simulink model "SESS_PassiveModel"  (R2018b)
settings: Solver=VariableStepAuto  StartTime=0.0  StopTime=1400  MaxStep=0.01  MinStep=0.00005  RelTol=1e-3
libraries: powerlib x4, electricdrivelib x1
settings Model: Creator=ttran  LastModifiedBy=ttran
settings SolverCC: ZeroCrossControl=EnableAll
settings DebuggingCC: IgnoredZcDiagnostic=none  SolverPrmCheckMsg=warning

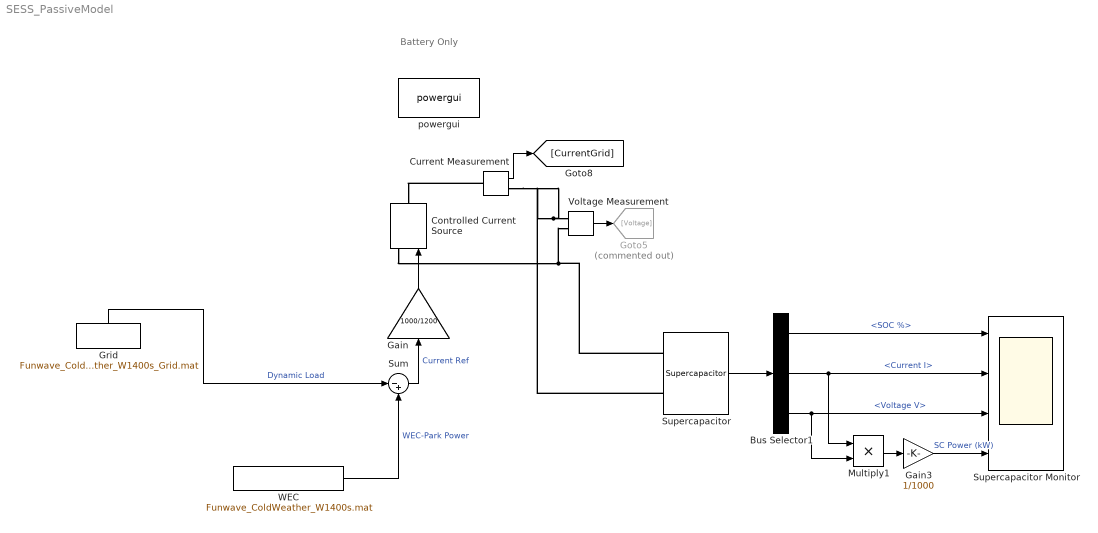
== system SESS_PassiveModel ==
  note: Battery Only
  Bus Selector1 : BusSelector  OutputSignals=SOC %,Current I,Voltage V
  Controlled Current Source : powerlib/Electrical Sources/Controlled Current Source  Initialize=on  Source_Type=AC  Amplitude=0  Phase=0  Frequency=0  Measurements=None
  Current Measurement : powerlib/Measurements/Current Measurement  PhasorSimulation=off  OutputType=Complex  PSBequivalent=0
  Gain : Gain  Gain=1000/1200
  Gain3 : Gain  Gain=1/1000
  Goto5 : Goto  Commented=on  GotoTag=Voltage
  Grid : FromFile  FileName=Funwave_ColdWeather_W1400s_Grid.mat  SampleTime=0
  Multiply1 : Product
  Sum : Sum  Inputs=|-+
  Supercapacitor : electricdrivelib/Extra Sources/Supercapacitor  C=1573  Rdc=8.9e-3  Voltage=380  Ns=144  Np=1  Vinit=340  Temp=25  PresetModel=off  EstParam=off  Nc=1  r=1e-9  epsilon=6.0208e-10  Ich=10  Vstern="[0.161  2.7  7.8]"  Self_dis=on  Ioc=10  Vself="[48  47.8  47.06  44.65]"  demandeplot=off  I="[10  20 100  500]"  Units=sec  Vmax=0  If=0  deltaV=0  alpha=0  sec=0
      settings: SourceProductName=Simscape Power Systems  SourceProductBaseCode=PS
  Supercapacitor Monitor : Scope  NumInputPorts=4
  Voltage Measurement : powerlib/Measurements/Voltage Measurement  PhasorSimulation=off  OutputType=Complex  PSBequivalent=0
  WEC : FromFile  FileName=Funwave_ColdWeather_W1400s.mat  SampleTime=0
  powergui : powerlib/powergui  Priority=1  SimulationMode=Continuous  SampleTime=50e-6  frequency=60  Iterations=50  frequencyindice=0  Pbase=100e6  ErrMax=1e-4  UnitsV=kV  UnitsW=MW  buscounter=0  FunctionMessages=off  echomessages=off  EnableUseOfTLC=off  CurrentSourceSwitches=off  DisableSnubberDevices=off  DisableRonSwitches=off  DisableVfSwitches=off  DisplayEquations=off  SolverType=Tustin/Backward Euler (TBE)  Interpol=off  ExternalGateDelay=off  methode=off  Ts=100  x0status=blocks  SPID=on  SwTol=0  HookPort=off  RestoreLinks=warning  ResistiveCurrentMeasurement=off  Frange=[0:2:500]  Ylog=off  Xlog=on  ShowGrid=off  save=off  variable=ZData  structure=0  ZoomFFT=off  StartTime=0.0  cycles=1  DisplayStyle=1  fundamental=60  FreqAxis=off  MaxFrequency=1000  frequencyindicesteady=1  RmsSteady=1  display=off
  wires:
  Voltage Measurement/1 -> Goto5/1
  Current Measurement/1 -> [CurrentGrid]
  Grid/1 -> Sum/1  "Dynamic Load"
  Bus Selector1/1 -> Supercapacitor Monitor/1  "<SOC %>"
  Bus Selector1/2 -> Supercapacitor Monitor/2, Multiply1/1  "<Current I>"
  Bus Selector1/3 -> Supercapacitor Monitor/3, Multiply1/2  "<Voltage V>"
  Multiply1/1 -> Gain3/1
  Supercapacitor/1 -> Bus Selector1/1
  Gain3/1 -> Supercapacitor Monitor/4  "SC Power (kW)"
  WEC/1 -> Sum/2  "WEC-Park Power"
  Gain/1 -> Controlled Current Source/1
  Sum/1 -> Gain/1  "Current Ref"
  connections:
  Supercapacitor/LConn2 -- Controlled Current Source/LConn1 -- Voltage Measurement/LConn2
  Current Measurement/LConn1 -- Controlled Current Source/RConn1
  Voltage Measurement/LConn1 -- Supercapacitor/LConn1 -- Current Measurement/RConn1
